simulink model "interp_with_preLookup_2D"  (R2017b)
settings: Solver=FixedStepAuto  StartTime=0.0  StopTime=10.0  FixedStep=0.1  RelTol=1e-3  EnableMultiTasking=on
settings Model: ExtModeAutoUpdateStatusClock=off  Creator=The MathWorks, Inc.  LastModifiedBy=hbourbou
settings DataIOCC: LimitDataPoints=on  SaveFormat=Array  SignalLoggingName=sigsOut
settings OptimizationCC: BooleanDataType=off  ExpressionDepthLimit=2147483647  InitFltsAndDblsToZero=on  LifeSpan=inf
settings DebuggingCC: SaveWithParameterizedLinksMsg=none  UnderspecifiedInitializationDetection=Classic  MergeDetectMultiDrivingBlocksExec=none  CheckExecutionContextPreStartOutputMsg=on  CheckExecutionContextRuntimeOutputMsg=on  SignalResolutionControl=TryResolveAllWithWarning  MultiTaskDSMMsg=warning  MultiTaskCondExecSysMsg=none  FcnCallInpInsideContextMsg=warning  StateNameClashWarn=warning  SFUnexpectedBacktrackingDiag=warning  SFNoUnconditionalDefaultTransitionDiag=warning  SFExecutionAtInitializationDiag=none
settings HardwareCC: ProdBitPerPointer=32  ProdBitPerSizeT=32  ProdBitPerPtrDiffT=32  ProdLargestAtomicFloat=None  ProdIntDivRoundTo=Undefined  ProdEndianess=Unspecified  ProdWordSize=32  ProdHWDeviceType=32-bit Generic  TargetUnknown=on
settings ModelReferenceCC: PropagateSignalLabelsOutOfModel=off
settings CodeAppCC: StateflowObjectComments=on
settings GRTTargetCC: TargetFcnLib=ansi_tfl_tmw.mat  TargetLangStandard=C89/C90 (ANSI)  GeneratePreprocessorConditionals=Disable all  CombineOutputUpdateFcns=off  GRTInterface=on
settings ConfigComp: CovMetricSettings=dw  CovHtmlReporting=on  CovSaveCumulativeToWorkspaceVar=on  CovSaveSingleToWorkspaceVar=on  CovExternalEMLEnable=off  CovSFcnEnable=off

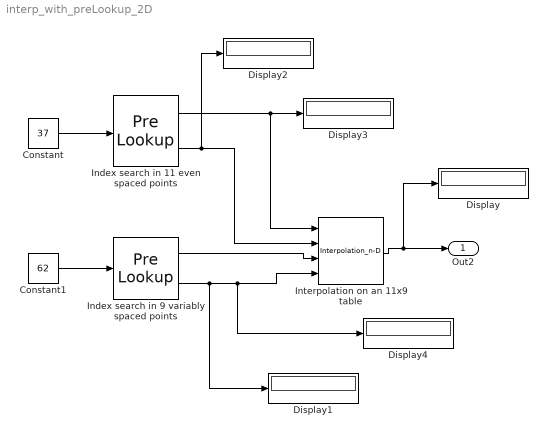
== system interp_with_preLookup_2D ==
  Constant : Constant  Value=37
  Constant1 : Constant  Value=62
  Display{,1..4} (5 alike) : Display
  Index search in 11 even spaced points : PreLookup  BreakpointsData=[0:10:100]  IndexSearchMethod=Evenly spaced points  ExtrapMethod=Linear
  Index search in 9 variably spaced points : PreLookup  BreakpointsData=[ 0.5, 1, 3, 5, 15, 45, 95, 96, 97 ]  BeginIndexSearchUsingPreviousIndexResult=on  ExtrapMethod=Linear
  Interpolation on an 11x9 table : Interpolation_n-D  Table=reshape([1:99], [11,9])  ExtrapMethod=Clip
  Out2 : Outport
  wires:
  Constant/1 -> Index search in 11 even spaced points/1
  Constant1/1 -> Index search in 9 variably spaced points/1
  Interpolation on an 11x9 table/1 -> Display/1, Out2/1
  Index search in 11 even spaced points/1 -> Display3/1, Interpolation on an 11x9 table/1
  Index search in 9 variably spaced points/1 -> Interpolation on an 11x9 table/3
  Index search in 9 variably spaced points/2 -> Display1/1, Interpolation on an 11x9 table/4, Display4/1
  Index search in 11 even spaced points/2 -> Display2/1, Interpolation on an 11x9 table/2
